simulink model "test_sliding_formation_gazebo_aerospace23a"  (R2023a)
settings: Solver=FixedStepAuto  StartTime=0.0  StopTime=inf  RelTol=1e-3
undefined symbols (not defined in the file or in its folder): angular, DiscIntNeverNeededParam, linear
libraries: ros2lib x11, simulink x4, robotcorelib x4
(part 1 of 2)
settings Model: Creator=johvany  LastModifiedBy=l15
settings OptimizationCC: EnhancedBackFolding=on  PassReuseOutputArgsThreshold=0  MaxStackSize=64  OptimizeBlockOrder=speed  DifferentSizesBufferReuse=on  OptimizationCustomize=off
settings DebuggingCC: ParameterTunabilityLossMsg=error
settings HardwareCC: ProdBitPerLong=64  ProdHWDeviceType=Intel->x86-64 (Linux 64)  UseEmbeddedCoderFeatures=off
settings SFSimCC: MATLABDynamicMemAlloc=off
settings RTWCC: Description=Simulink Desktop Real-Time  SystemTargetFile=sldrt.tlc  TemplateMakefile=sldrt.tmf  Toolchain=Colcon Tools  RTWCompilerOptimization=on
settings CodeAppCC: ForceParamTrailComments=on  MaxIdLength=95  OperatorAnnotations=on
settings SimulinkDesktopRealTimeCC: TargetLibSuffix=_sldrt.a  TargetPreCompLibLocation=/usr/local/MATLAB/R2023b/toolbox/sldrt/lib/glnxa64  TargetLangStandard=C89/C90 (ANSI)

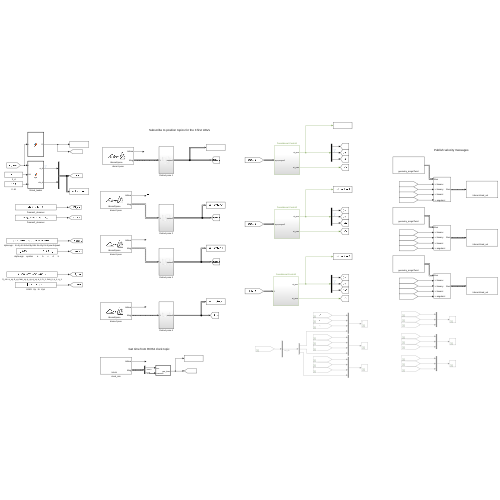
[thumbnail: Simulink's stored preview of the top-level diagram]
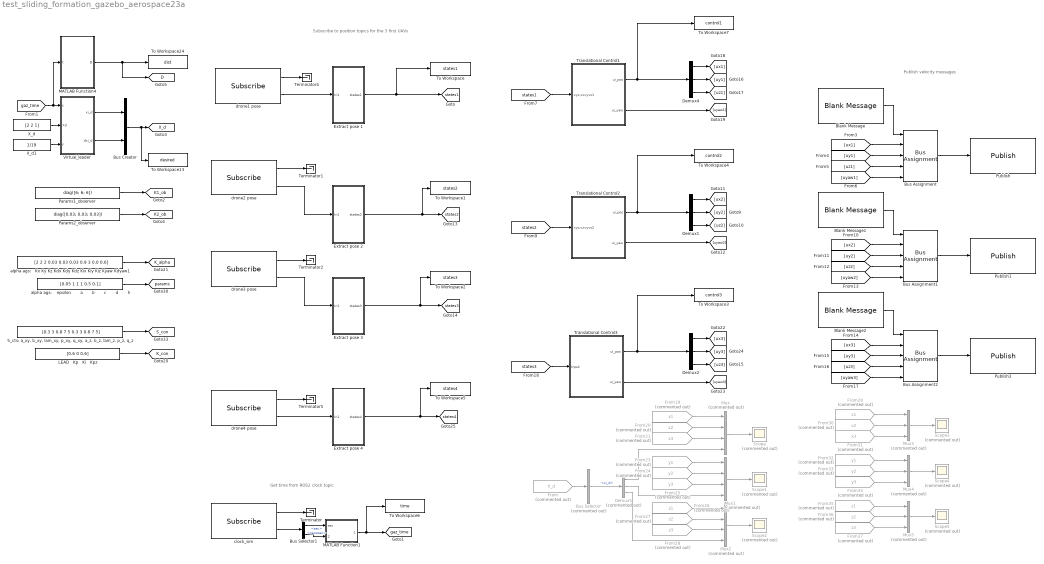
== system test_sliding_formation_gazebo_aerospace23a ==
  note: Publish velocity messages
  note: Subscribe to position topics for the 3 first UAVs
  note: Get time from ROS2 clock topic
  Blank Message : ros2lib/Blank Message  messageClass=Message  entityType=geometry_msgs/Twist  messageType=geometry_msgs/Twist  SampleTime=inf
  Blank Message1 : ros2lib/Blank Message  messageClass=Message  entityType=geometry_msgs/Twist  messageType=geometry_msgs/Twist  SampleTime=inf
  Blank Message2 : ros2lib/Blank Message  messageClass=Message  entityType=geometry_msgs/Twist  messageType=geometry_msgs/Twist  SampleTime=inf
  Bus Assignment : BusAssignment  AssignedSignals=linear.x,linear.y,linear.z,angular.z
  Bus Assignment1 : BusAssignment  AssignedSignals=linear.x,linear.y,linear.z,angular.z
  Bus Assignment2 : BusAssignment  AssignedSignals=linear.x,linear.y,linear.z,angular.z
  Bus Creator : BusCreator  Inputs=2
  Bus Selector : BusSelector  Commented=on  OutputSignals=xi_d
  Bus Selector1 : BusSelector  OutputSignals=clock.sec,clock.nanosec
  Demux1 : Demux  Outputs=3
  Demux2 : Demux  Outputs=3
  Demux4 : Demux  Outputs=3
  Demux5 : Demux  Commented=on  Outputs=3
  Extract pose 1 : Subsystem
  Extract pose 2 : Subsystem
  Extract pose 3 : Subsystem
  Extract pose 4 : Subsystem
  From : From  Commented=on  GotoTag=X_d  TagVisibility=global
      settings: CloseFcn=tagdialog Close
  From19 : From  Commented=on  GotoTag=x1  TagVisibility=global
      settings: CloseFcn=tagdialog Close
  From20 : From  Commented=on  GotoTag=x2  TagVisibility=global
      settings: CloseFcn=tagdialog Close
  From21 : From  Commented=on  GotoTag=x3  TagVisibility=global
      settings: CloseFcn=tagdialog Close
  From23 : From  Commented=on  GotoTag=y1  TagVisibility=global
      settings: CloseFcn=tagdialog Close
  From24 : From  Commented=on  GotoTag=y2  TagVisibility=global
      settings: CloseFcn=tagdialog Close
  From25 : From  Commented=on  GotoTag=y3  TagVisibility=global
      settings: CloseFcn=tagdialog Close
  From26 : From  Commented=on  GotoTag=z1  TagVisibility=global
      settings: CloseFcn=tagdialog Close
  From27 : From  Commented=on  GotoTag=z2  TagVisibility=global
      settings: CloseFcn=tagdialog Close
  From28 : From  Commented=on  GotoTag=z3  TagVisibility=global
      settings: CloseFcn=tagdialog Close
  From29 : From  Commented=on  GotoTag=x1  TagVisibility=global
      settings: CloseFcn=tagdialog Close
  From30 : From  Commented=on  GotoTag=x2  TagVisibility=global
      settings: CloseFcn=tagdialog Close
  From31 : From  Commented=on  GotoTag=x3  TagVisibility=global
      settings: CloseFcn=tagdialog Close
  From32 : From  Commented=on  GotoTag=y1  TagVisibility=global
      settings: CloseFcn=tagdialog Close
  From33 : From  Commented=on  GotoTag=y2  TagVisibility=global
      settings: CloseFcn=tagdialog Close
  From34 : From  Commented=on  GotoTag=y3  TagVisibility=global
      settings: CloseFcn=tagdialog Close
  From35 : From  Commented=on  GotoTag=z1  TagVisibility=global
      settings: CloseFcn=tagdialog Close
  From36 : From  Commented=on  GotoTag=z2  TagVisibility=global
      settings: CloseFcn=tagdialog Close
  From37 : From  Commented=on  GotoTag=z3  TagVisibility=global
      settings: CloseFcn=tagdialog Close
  LEAD   Kp   Ki   Kpz : Constant  Value=[0.6 0 0.6]
  MATLAB Function1 : MATLAB Function  TreatAsAtomicUnit=on
  MATLAB Function4 : MATLAB Function  TreatAsAtomicUnit=on
  Mux : Mux  Commented=on
  Mux1 : Mux  Commented=on
  Mux2 : Mux  Commented=on
  Mux3 : Mux  Commented=on  Inputs=3
  Mux4 : Mux  Commented=on  Inputs=3
  Mux5 : Mux  Commented=on  Inputs=3
  Params1_observer : Constant  Value=diag([6; 6; 6])
  Params2_observer : Constant  Value=diag([0.03; 0.03; 0.03])
  Publish : ros2lib/Publish  topicSource=Select from ROS network  topic=/drone1/cmd_vel  messageType=geometry_msgs/Twist  QOSHistory=Keep last  QOSDepth=1  QOSReliability=Reliable  QOSDurability=Volatile
  Publish1 : ros2lib/Publish  topicSource=Select from ROS network  topic=/drone2/cmd_vel  messageType=geometry_msgs/Twist  QOSHistory=Keep last  QOSDepth=1  QOSReliability=Reliable  QOSDurability=Volatile
  Publish2 : ros2lib/Publish  topicSource=Select from ROS network  topic=/drone3/cmd_vel  messageType=geometry_msgs/Twist  QOSHistory=Keep last  QOSDepth=1  QOSReliability=Reliable  QOSDurability=Volatile
  "S_cts: a_xy, b_xy, lam_xy, p_xy, q_xy, a_z, b_z, lam_z, p_z, q_z" : Constant  Value=[0.3 3 0.8 7 5 0.3 3 0.8 7 5]
  Scope{,1..5} (6 alike) : Scope  Commented=on
  Terminator{,1..2,4..5} (5 alike) : Terminator
  To Workspace : ToWorkspace  VariableName=states1  SampleTime=-1
  To Workspace1 : ToWorkspace  VariableName=states2  SampleTime=-1
  To Workspace13 : ToWorkspace  VariableName=desired  SampleTime=-1
  To Workspace2 : ToWorkspace  VariableName=states3  SampleTime=-1
  To Workspace24 : ToWorkspace  VariableName=dist  SampleTime=-1
  To Workspace3 : ToWorkspace  VariableName=control3  SampleTime=-1
  To Workspace4 : ToWorkspace  VariableName=control2  SampleTime=-1
  To Workspace5 : ToWorkspace  VariableName=states4  SampleTime=-1
  To Workspace6 : ToWorkspace  VariableName=time  SampleTime=-1
  To Workspace7 : ToWorkspace  VariableName=control1  SampleTime=-1
  Translational Control1 : Subsystem
  Translational Control2 : Subsystem
  Translational Control3 : Subsystem
  Virtual_leader : MATLAB Function  TreatAsAtomicUnit=on
  X_d : Constant  Value=[2 2 1]
  X_d1 : Constant  Value=1/19
  alpha ags:    epsilon       a       b       c       d       h : Constant  Value=[0.05 1 1 1 0.5 0.1]
  alpha ags:   Kx Ky Kz Kdx Kdy Kdz Kix Kiy Kiz Kyaw Kdyaw1 : Constant  Value=[2 2 2 0.03 0.03 0.03 0.9 3 0.0 0.6]
  clock_sim : ros2lib/Subscribe  topicSource=Select from ROS network  topic=/clock  messageType=rosgraph_msgs/Clock  sampleTime=-1  QOSHistory=Keep last  QOSDepth=1  QOSReliability=Reliable  QOSDurability=Volatile
  drone1 pose : ros2lib/Subscribe  topicSource=Select from ROS network  topic=/drone1/pose  messageType=geometry_msgs/PoseStamped  sampleTime=-1  QOSHistory=Keep last  QOSDepth=1  QOSReliability=Reliable  QOSDurability=Volatile
  drone2 pose : ros2lib/Subscribe  topicSource=Select from ROS network  topic=/drone2/pose  messageType=geometry_msgs/PoseStamped  sampleTime=-1  QOSHistory=Keep last  QOSDepth=1  QOSReliability=Reliable  QOSDurability=Volatile
  drone3 pose : ros2lib/Subscribe  topicSource=Select from ROS network  topic=/drone3/pose  messageType=geometry_msgs/PoseStamped  sampleTime=-1  QOSHistory=Keep last  QOSDepth=1  QOSReliability=Reliable  QOSDurability=Volatile
  drone4 pose : ros2lib/Subscribe  topicSource=Select from ROS network  topic=/drone4/pose  messageType=geometry_msgs/PoseStamped  sampleTime=-1  QOSHistory=Keep last  QOSDepth=1  QOSReliability=Reliable  QOSDurability=Volatile
  tag scope: D=global, K1_ob=global, K2_ob=global, K_alpha=global, K_con=global, S_con=global, X_d=global, gaz_time=global, params=global, states1=global, states2=global, states3=global, states4=global
  wires:
  clock_sim/1 -> Terminator/1
  drone2 pose/2 -> Extract pose 2/1(In1)
  drone2 pose/1 -> Terminator1/1
  drone3 pose/2 -> Extract pose 3/1(In1)
  drone3 pose/1 -> Terminator2/1
  Blank Message/1 -> Bus Assignment/1
  Bus Assignment/1 -> Publish/1
  Blank Message1/1 -> Bus Assignment1/1
  Bus Assignment1/1 -> Publish1/1
  Blank Message2/1 -> Bus Assignment2/1
  Bus Assignment2/1 -> Publish2/1
  clock_sim/2 -> Bus Selector1/1
  Bus Selector1/1 -> MATLAB Function1/1(sec)  "<sec>"
  Bus Selector1/2 -> MATLAB Function1/2(nanosec)  "<nanosec>"
  Virtual_leader/2(dxi_d) -> Bus Creator/2
  Bus Creator/1 -> To Workspace13/1, [X_d]
  Virtual_leader/1(xi_d) -> Bus Creator/1
  drone1 pose/1 -> Terminator4/1
  drone1 pose/2 -> Extract pose 1/1(In1)
  MATLAB Function1/1(gaz_time) -> To Workspace6/1, [gaz_time]
  Extract pose 1/1(states1) -> To Workspace/1, [states1]
  [ux1] -> Bus Assignment/2
  [uy1] -> Bus Assignment/3
  [uz1] -> Bus Assignment/4
  [uyaw1] -> Bus Assignment/5
  X_d/1 -> Virtual_leader/2(Xd)
  Extract pose 2/1(states2) -> To Workspace1/1, [states2]
  Extract pose 3/1(states3) -> To Workspace2/1, [states3]
  [ux2] -> Bus Assignment1/2
  [uy2] -> Bus Assignment1/3
  [uz2] -> Bus Assignment1/4
  [uyaw2] -> Bus Assignment1/5
  [uy3] -> Bus Assignment2/3
  [uyaw3] -> Bus Assignment2/5
  [uz3] -> Bus Assignment2/4
  [ux3] -> Bus Assignment2/2
  Translational Control1/2(ui_yaw) -> [uyaw1]
  Demux4/2 -> [uy1]
  Demux4/3 -> [uz1]
  [states1] -> Translational Control1/1(xyz,vxvyvz1)
  Demux4/1 -> [ux1]
  LEAD   Kp   Ki   Kpz/1 -> [K_con]
  alpha ags:   Kx Ky Kz Kdx Kdy Kdz Kix Kiy Kiz Kyaw Kdyaw1/1 -> [K_alpha]
  alpha ags:    epsilon       a       b       c       d       h/1 -> [params]
  X_d1/1 -> Virtual_leader/3(f)
  "S_cts: a_xy, b_xy, lam_xy, p_xy, q_xy, a_z, b_z, lam_z, p_z, q_z"/1 -> [S_con]
  MATLAB Function4/1(D) -> [D], To Workspace24/1
  [gaz_time] -> MATLAB Function4/1(t), Virtual_leader/1(t)
  Translational Control1/1(ui_pos) -> Demux4/1, To Workspace7/1
  Params1_observer/1 -> [K1_ob]
  Params2_observer/1 -> [K2_ob]
  Translational Control2/1(ui_pos) -> Demux1/1, To Workspace4/1
  Demux1/1 -> [ux2]
  [states2] -> Translational Control2/1(xyz,vxvyvz2)
  Demux1/3 -> [uz2]
  Demux1/2 -> [uy2]
  Translational Control2/2(ui_yaw) -> [uyaw2]
  Translational Control3/2(ui_yaw) -> [uyaw3]
  Demux2/2 -> [uy3]
  Demux2/3 -> [uz3]
  [states3] -> Translational Control3/1(Input)
  Demux2/1 -> [ux3]
  Translational Control3/1(ui_pos) -> Demux2/1, To Workspace3/1
  Extract pose 4/1(states4) -> [states4], To Workspace5/1
  drone4 pose/1 -> Terminator5/1
  drone4 pose/2 -> Extract pose 4/1(In1)
  From19/1 -> Mux/1
  From20/1 -> Mux/2
  From21/1 -> Mux/3
  Mux/1 -> Scope/1
  Bus Selector/1 -> Demux5/1  "<xi_d>"
  From/1 -> Bus Selector/1
  Demux5/1 -> Mux/4
  Demux5/2 -> Mux1/4
  Mux1/1 -> Scope1/1
  From25/1 -> Mux1/3
  From24/1 -> Mux1/2
  From23/1 -> Mux1/1
  From26/1 -> Mux2/1
  From27/1 -> Mux2/2
  From28/1 -> Mux2/3
  Mux2/1 -> Scope2/1
  Demux5/3 -> Mux2/4
  Mux5/1 -> Scope5/1
  From37/1 -> Mux5/3
  From36/1 -> Mux5/2
  From35/1 -> Mux5/1
  From32/1 -> Mux4/1
  From33/1 -> Mux4/2
  From34/1 -> Mux4/3
  Mux4/1 -> Scope4/1
  Mux3/1 -> Scope3/1
  From31/1 -> Mux3/3
  From30/1 -> Mux3/2
  From29/1 -> Mux3/1

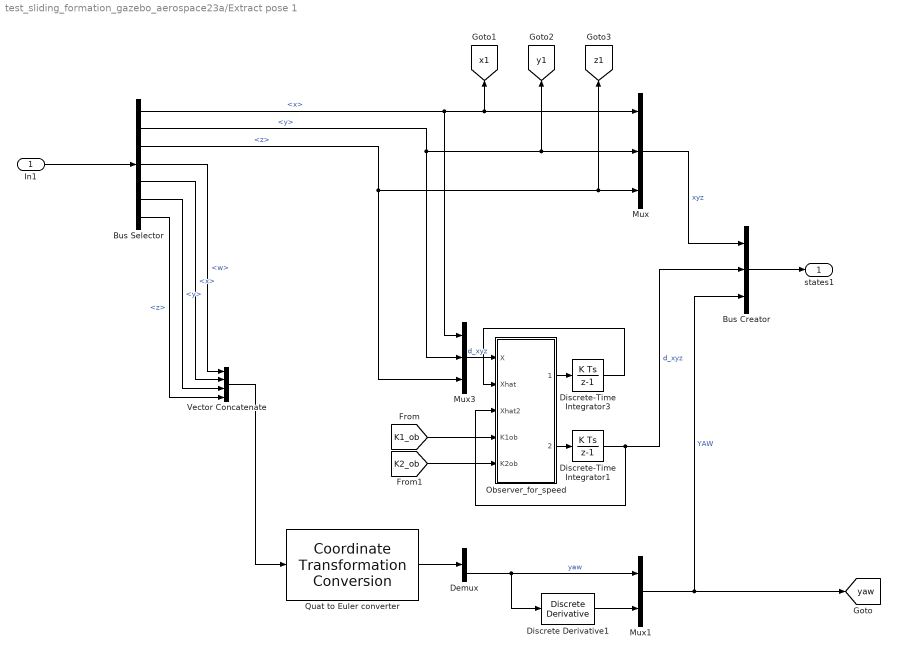
== system test_sliding_formation_gazebo_aerospace23a/Extract pose 1 ==
  In1 : Inport
  Bus Creator : BusCreator  Inputs=3
  Bus Selector : BusSelector  OutputSignals=pose.position.x,pose.position.y,pose.position.z,pose.orientation.w,pose.orientation.x,pose.orientation.y,pose.orientation.z
  Demux : Demux  Outputs=3
  Discrete Derivative1 : simulink/Discrete/Discrete Derivative  gainval=1.0  ICPrevScaledInput=0.0  OutMin=[]  OutMax=[]  OutDataType=fixdt(1, 16)  OutScaling=2^-10  DoSatur=off
  Discrete-Time Integrator1 : DiscreteIntegrator  SampleTime=-1  UpperSaturationLimit=1  LowerSaturationLimit=-1  ICPrevOutput=DiscIntNeverNeededParam  ICPrevScaledInput=DiscIntNeverNeededParam
  Discrete-Time Integrator3 : DiscreteIntegrator  SampleTime=-1  UpperSaturationLimit=1  LowerSaturationLimit=-1  ICPrevOutput=DiscIntNeverNeededParam  ICPrevScaledInput=DiscIntNeverNeededParam
  Mux : Mux  Inputs=3
  Mux1 : Mux  Inputs=2
  Mux3 : Mux  Inputs=3
  Observer_for_speed : MATLAB Function  TreatAsAtomicUnit=on
  Quat to Euler converter : robotcorelib/Coordinate Transformation Conversion  InputRepresentation=Quaternion  InputEulerSequence=ZYX  ShowTrVecInputPort=on  OutputRepresentation=Euler Angles  OutputEulerSequence=XYZ  ShowTrVecOutputPort=on  SimulateUsing=Interpreted execution
      settings: LibrarySourceBlock=roslib/Utilities/Coordinate Transformation Conversion
  Vector Concatenate : Concatenate  NumInputs=4
  states1 : Outport
  tag scope: x1=global, y1=global, yaw=global, z1=global
  wires:
  Bus Selector/5 -> Vector Concatenate/2  "<x>"
  Quat to Euler converter/1 -> Demux/1
  Bus Selector/6 -> Vector Concatenate/3  "<y>"
  Bus Selector/7 -> Vector Concatenate/4  "<z>"
  Vector Concatenate/1 -> Quat to Euler converter/1
  In1/1 -> Bus Selector/1
  Bus Selector/4 -> Vector Concatenate/1  "<w>"
  Demux/3 -> Discrete Derivative1/1, Mux1/1  "yaw"
  Mux/1 -> Bus Creator/1  "xyz"
  Bus Creator/1 -> states1/1
  Discrete Derivative1/1 -> Mux1/2
  Bus Selector/3 -> Mux3/3, [z1], Mux/3  "<z>"
  Bus Selector/2 -> Mux3/2, [y1], Mux/2  "<y>"
  Bus Selector/1 -> Mux3/1, [x1], Mux/1  "<x>"
  Mux1/1 -> [yaw], Bus Creator/3  "YAW"
  Discrete-Time Integrator1/1 -> Observer_for_speed/3(Xhat2), Bus Creator/2  "d_xyz"
  Discrete-Time Integrator3/1 -> Observer_for_speed/2(Xhat)
  Observer_for_speed/1(dXhat_1) -> Discrete-Time Integrator3/1
  Observer_for_speed/2(dXhat_2) -> Discrete-Time Integrator1/1
  Mux3/1 -> Observer_for_speed/1(X)  "d_xyz"
  [K1_ob] -> Observer_for_speed/4(K1ob)
  [K2_ob] -> Observer_for_speed/5(K2ob)

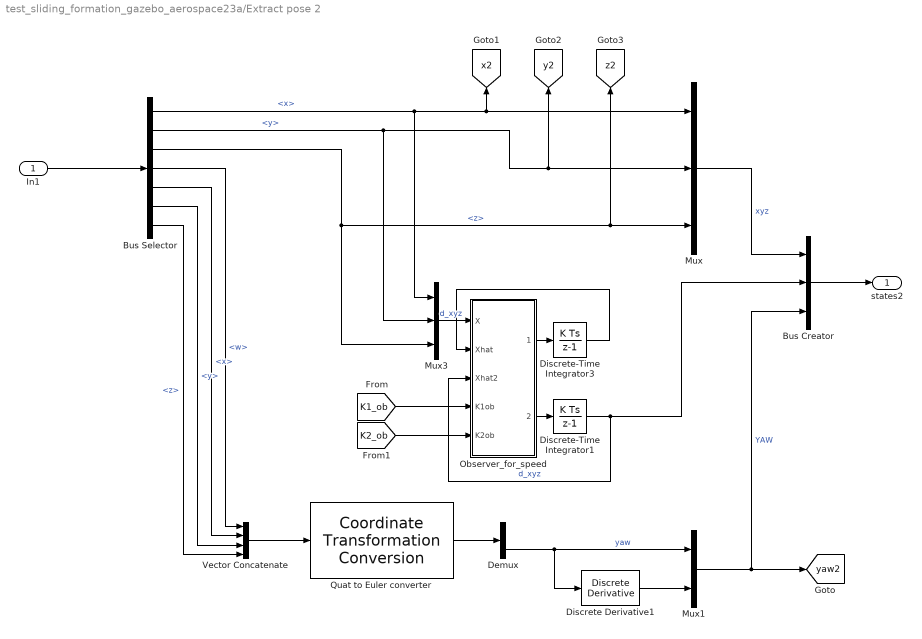
== system test_sliding_formation_gazebo_aerospace23a/Extract pose 2 ==
  In1 : Inport
  Bus Creator : BusCreator  Inputs=3
  Bus Selector : BusSelector  OutputSignals=pose.position.x,pose.position.y,pose.position.z,pose.orientation.w,pose.orientation.x,pose.orientation.y,pose.orientation.z
  Demux : Demux  Outputs=3
  Discrete Derivative1 : simulink/Discrete/Discrete Derivative  gainval=1.0  ICPrevScaledInput=0.0  OutMin=[]  OutMax=[]  OutDataType=fixdt(1, 16)  OutScaling=2^-10  DoSatur=off
  Discrete-Time Integrator1 : DiscreteIntegrator  SampleTime=-1  UpperSaturationLimit=1  LowerSaturationLimit=-1  ICPrevOutput=DiscIntNeverNeededParam  ICPrevScaledInput=DiscIntNeverNeededParam
  Discrete-Time Integrator3 : DiscreteIntegrator  SampleTime=-1  UpperSaturationLimit=1  LowerSaturationLimit=-1  ICPrevOutput=DiscIntNeverNeededParam  ICPrevScaledInput=DiscIntNeverNeededParam
  Mux : Mux  Inputs=3
  Mux1 : Mux  Inputs=2
  Mux3 : Mux  Inputs=3
  Observer_for_speed : MATLAB Function  TreatAsAtomicUnit=on
  Quat to Euler converter : robotcorelib/Coordinate Transformation Conversion  InputRepresentation=Quaternion  InputEulerSequence=ZYX  ShowTrVecInputPort=on  OutputRepresentation=Euler Angles  OutputEulerSequence=XYZ  ShowTrVecOutputPort=on  SimulateUsing=Interpreted execution
      settings: LibrarySourceBlock=roslib/Utilities/Coordinate Transformation Conversion
  Vector Concatenate : Concatenate  NumInputs=4
  states2 : Outport
  tag scope: x2=global, y2=global, yaw2=global, z2=global
  wires:
  Discrete Derivative1/1 -> Mux1/2
  Bus Creator/1 -> states2/1
  Mux/1 -> Bus Creator/1  "xyz"
  Demux/3 -> Discrete Derivative1/1, Mux1/1  "yaw"
  Bus Selector/4 -> Vector Concatenate/1  "<w>"
  In1/1 -> Bus Selector/1
  Vector Concatenate/1 -> Quat to Euler converter/1
  Bus Selector/7 -> Vector Concatenate/4  "<z>"
  Bus Selector/6 -> Vector Concatenate/3  "<y>"
  Quat to Euler converter/1 -> Demux/1
  Bus Selector/5 -> Vector Concatenate/2  "<x>"
  Mux3/1 -> Observer_for_speed/1(X)  "d_xyz"
  Observer_for_speed/1(dXhat_1) -> Discrete-Time Integrator3/1
  Observer_for_speed/2(dXhat_2) -> Discrete-Time Integrator1/1
  [K1_ob] -> Observer_for_speed/4(K1ob)
  Bus Selector/2 -> Mux3/2, [y2], Mux/2  "<y>"
  Bus Selector/1 -> Mux3/1, [x2], Mux/1  "<x>"
  Discrete-Time Integrator3/1 -> Observer_for_speed/2(Xhat)
  Discrete-Time Integrator1/1 -> Bus Creator/2, Observer_for_speed/3(Xhat2)  "d_xyz"
  [K2_ob] -> Observer_for_speed/5(K2ob)
  Bus Selector/3 -> Mux3/3, [z2], Mux/3  "<z>"
  Mux1/1 -> [yaw2], Bus Creator/3  "YAW"

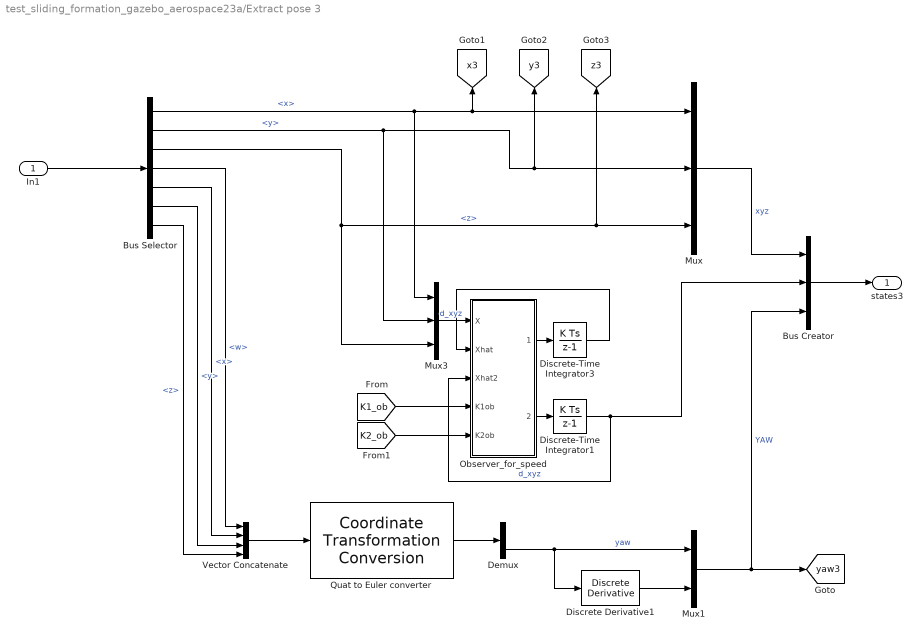
== system test_sliding_formation_gazebo_aerospace23a/Extract pose 3 ==
  In1 : Inport
  Bus Creator : BusCreator  Inputs=3
  Bus Selector : BusSelector  OutputSignals=pose.position.x,pose.position.y,pose.position.z,pose.orientation.w,pose.orientation.x,pose.orientation.y,pose.orientation.z
  Demux : Demux  Outputs=3
  Discrete Derivative1 : simulink/Discrete/Discrete Derivative  gainval=1.0  ICPrevScaledInput=0.0  OutMin=[]  OutMax=[]  OutDataType=fixdt(1, 16)  OutScaling=2^-10  DoSatur=off
  Discrete-Time Integrator1 : DiscreteIntegrator  SampleTime=-1  UpperSaturationLimit=1  LowerSaturationLimit=-1  ICPrevOutput=DiscIntNeverNeededParam  ICPrevScaledInput=DiscIntNeverNeededParam
  Discrete-Time Integrator3 : DiscreteIntegrator  SampleTime=-1  UpperSaturationLimit=1  LowerSaturationLimit=-1  ICPrevOutput=DiscIntNeverNeededParam  ICPrevScaledInput=DiscIntNeverNeededParam
  Mux : Mux  Inputs=3
  Mux1 : Mux  Inputs=2
  Mux3 : Mux  Inputs=3
  Observer_for_speed : MATLAB Function  TreatAsAtomicUnit=on
  Quat to Euler converter : robotcorelib/Coordinate Transformation Conversion  InputRepresentation=Quaternion  InputEulerSequence=ZYX  ShowTrVecInputPort=on  OutputRepresentation=Euler Angles  OutputEulerSequence=XYZ  ShowTrVecOutputPort=on  SimulateUsing=Interpreted execution
      settings: LibrarySourceBlock=roslib/Utilities/Coordinate Transformation Conversion
  Vector Concatenate : Concatenate  NumInputs=4
  states3 : Outport
  tag scope: x3=global, y3=global, yaw3=global, z3=global
  wires:
  Mux1/1 -> Bus Creator/3, [yaw3]  "YAW"
  Bus Selector/3 -> [z3], Mux/3, Mux3/3  "<z>"
  [K2_ob] -> Observer_for_speed/5(K2ob)
  Discrete-Time Integrator1/1 -> Observer_for_speed/3(Xhat2), Bus Creator/2  "d_xyz"
  Discrete-Time Integrator3/1 -> Observer_for_speed/2(Xhat)
  Bus Selector/1 -> [x3], Mux/1, Mux3/1  "<x>"
  Bus Selector/2 -> [y3], Mux/2, Mux3/2  "<y>"
  [K1_ob] -> Observer_for_speed/4(K1ob)
  Observer_for_speed/2(dXhat_2) -> Discrete-Time Integrator1/1
  Observer_for_speed/1(dXhat_1) -> Discrete-Time Integrator3/1
  Mux3/1 -> Observer_for_speed/1(X)  "d_xyz"
  Bus Selector/5 -> Vector Concatenate/2  "<x>"
  Quat to Euler converter/1 -> Demux/1
  Bus Selector/6 -> Vector Concatenate/3  "<y>"
  Bus Selector/7 -> Vector Concatenate/4  "<z>"
  Vector Concatenate/1 -> Quat to Euler converter/1
  In1/1 -> Bus Selector/1
  Bus Selector/4 -> Vector Concatenate/1  "<w>"
  Demux/3 -> Mux1/1, Discrete Derivative1/1  "yaw"
  Mux/1 -> Bus Creator/1  "xyz"
  Bus Creator/1 -> states3/1
  Discrete Derivative1/1 -> Mux1/2

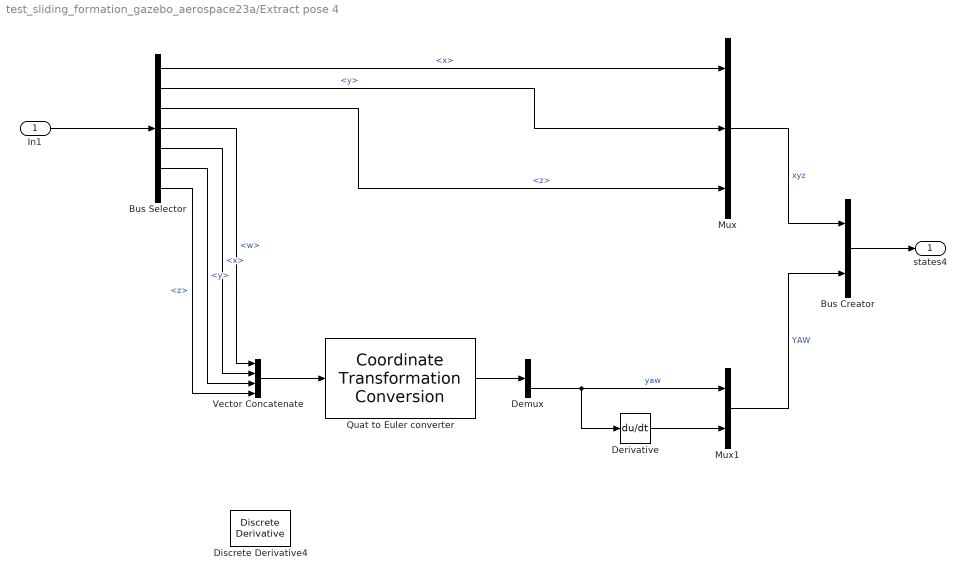
== system test_sliding_formation_gazebo_aerospace23a/Extract pose 4 ==
  In1 : Inport
  Bus Creator : BusCreator  Inputs=2
  Bus Selector : BusSelector  OutputSignals=pose.position.x,pose.position.y,pose.position.z,pose.orientation.w,pose.orientation.x,pose.orientation.y,pose.orientation.z
  Demux : Demux  Outputs=3
  Derivative : Derivative
  Discrete Derivative4 : simulink/Discrete/Discrete Derivative  gainval=1.0  ICPrevScaledInput=0.0  OutMin=[]  OutMax=[]  OutDataType=fixdt(1, 16)  OutScaling=2^-10  DoSatur=off
  Mux : Mux  Inputs=3
  Mux1 : Mux  Inputs=2
  Quat to Euler converter : robotcorelib/Coordinate Transformation Conversion  InputRepresentation=Quaternion  InputEulerSequence=ZYX  ShowTrVecInputPort=on  OutputRepresentation=Euler Angles  OutputEulerSequence=XYZ  ShowTrVecOutputPort=on  SimulateUsing=Interpreted execution
      settings: LibrarySourceBlock=roslib/Utilities/Coordinate Transformation Conversion
  Vector Concatenate : Concatenate  NumInputs=4
  states4 : Outport
  wires:
  Bus Selector/5 -> Vector Concatenate/2  "<x>"
  Quat to Euler converter/1 -> Demux/1
  Bus Selector/6 -> Vector Concatenate/3  "<y>"
  Bus Selector/1 -> Mux/1  "<x>"
  Bus Selector/7 -> Vector Concatenate/4  "<z>"
  Vector Concatenate/1 -> Quat to Euler converter/1
  In1/1 -> Bus Selector/1
  Bus Selector/4 -> Vector Concatenate/1  "<w>"
  Bus Selector/2 -> Mux/2  "<y>"
  Bus Selector/3 -> Mux/3  "<z>"
  Demux/3 -> Derivative/1, Mux1/1  "yaw"
  Mux/1 -> Bus Creator/1  "xyz"
  Bus Creator/1 -> states4/1
  Derivative/1 -> Mux1/2
  Mux1/1 -> Bus Creator/2  "YAW"

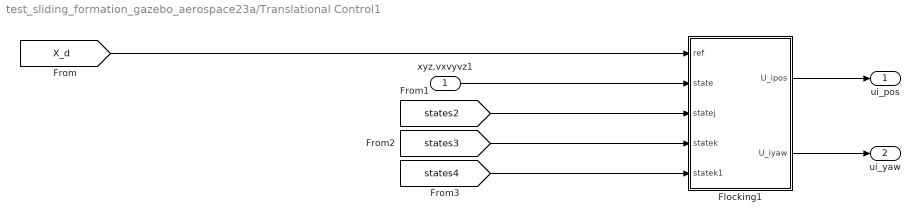
== system test_sliding_formation_gazebo_aerospace23a/Translational Control1 ==
  xyz,vxvyvz1 : Inport
  Flocking1 : Subsystem
  ui_pos : Outport  VectorParamsAs1DForOutWhenUnconnected=off
  ui_yaw : Outport  Port=2  VectorParamsAs1DForOutWhenUnconnected=off
  wires:
  [states2] -> Flocking1/3(statej)
  [states3] -> Flocking1/4(statek)
  [states4] -> Flocking1/5(statek1)
  Flocking1/1(U_ipos) -> ui_pos/1
  Flocking1/2(U_iyaw) -> ui_yaw/1
  [X_d] -> Flocking1/1(ref)
  xyz,vxvyvz1/1 -> Flocking1/2(state)

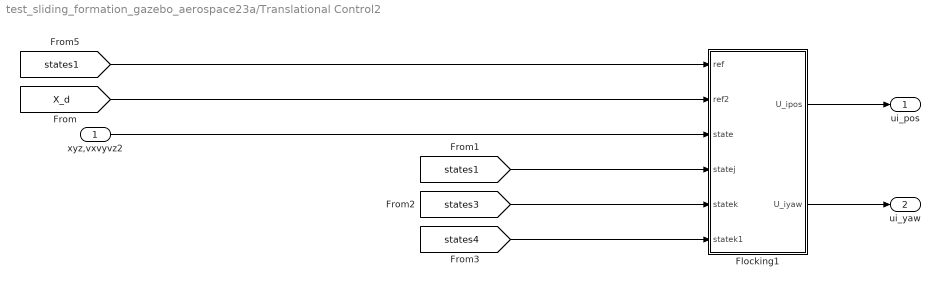
== system test_sliding_formation_gazebo_aerospace23a/Translational Control2 ==
  xyz,vxvyvz2 : Inport
  Flocking1 : Subsystem
  ui_pos : Outport  VectorParamsAs1DForOutWhenUnconnected=off
  ui_yaw : Outport  Port=2  VectorParamsAs1DForOutWhenUnconnected=off
  wires:
  Flocking1/2(U_iyaw) -> ui_yaw/1
  Flocking1/1(U_ipos) -> ui_pos/1
  [states4] -> Flocking1/6(statek1)
  [states3] -> Flocking1/5(statek)
  [states1] -> Flocking1/4(statej)
  [states1] -> Flocking1/1(ref)
  [X_d] -> Flocking1/2(ref2)
  xyz,vxvyvz2/1 -> Flocking1/3(state)

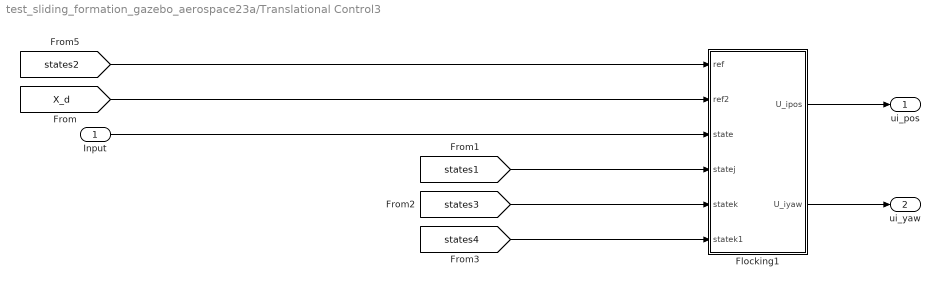
== system test_sliding_formation_gazebo_aerospace23a/Translational Control3 ==
  Input : Inport
  Flocking1 : Subsystem
  ui_pos : Outport  VectorParamsAs1DForOutWhenUnconnected=off
  ui_yaw : Outport  Port=2  VectorParamsAs1DForOutWhenUnconnected=off
  wires:
  [X_d] -> Flocking1/2(ref2)
  [states2] -> Flocking1/1(ref)
  [states1] -> Flocking1/4(statej)
  [states3] -> Flocking1/5(statek)
  [states4] -> Flocking1/6(statek1)
  Flocking1/1(U_ipos) -> ui_pos/1
  Flocking1/2(U_iyaw) -> ui_yaw/1
  Input/1 -> Flocking1/3(state)

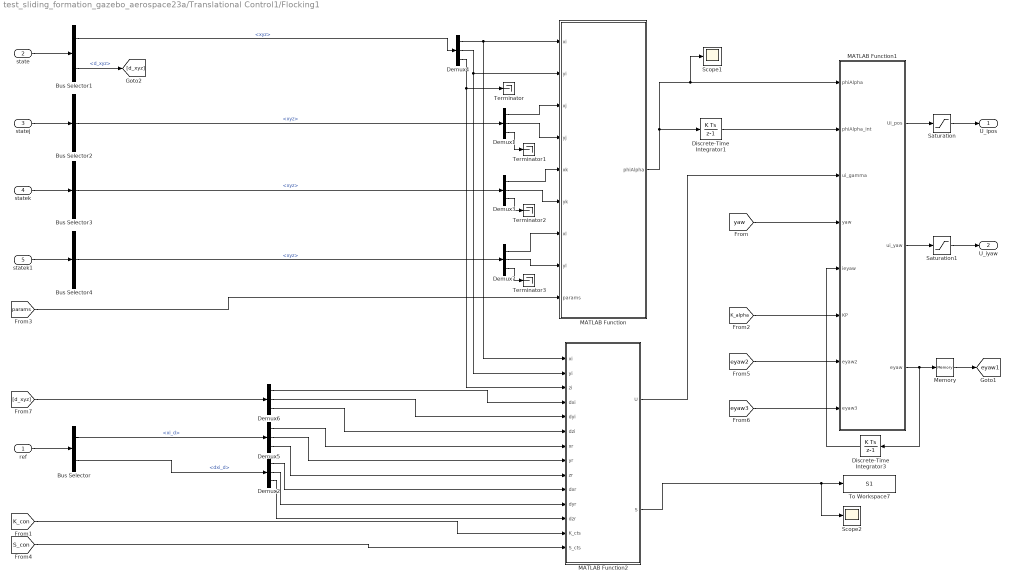
== system test_sliding_formation_gazebo_aerospace23a/Translational Control1/Flocking1 ==
  ref : Inport
  state : Inport  Port=2
  statej : Inport  Port=3
  statek : Inport  Port=4
  statek1 : Inport  Port=5
  Bus Selector : BusSelector  OutputSignals=xi_d,dxi_d
  Bus Selector1 : BusSelector  OutputSignals=xyz,d_xyz
  Bus Selector2 : BusSelector  OutputSignals=xyz
  Bus Selector3 : BusSelector  OutputSignals=xyz
  Bus Selector4 : BusSelector  OutputSignals=xyz
  Demux{1..7} (7 alike) : Demux  Outputs=3
  Discrete-Time Integrator1 : DiscreteIntegrator  SampleTime=-1  LimitOutput=on  UpperSaturationLimit=5  LowerSaturationLimit=-5  ICPrevOutput=DiscIntNeverNeededParam  ICPrevScaledInput=DiscIntNeverNeededParam
  Discrete-Time Integrator3 : DiscreteIntegrator  SampleTime=-1  LimitOutput=on  UpperSaturationLimit=1  LowerSaturationLimit=-1  ICPrevOutput=DiscIntNeverNeededParam  ICPrevScaledInput=DiscIntNeverNeededParam
  MATLAB Function : MATLAB Function  TreatAsAtomicUnit=on
  MATLAB Function1 : MATLAB Function  TreatAsAtomicUnit=on
  MATLAB Function2 : MATLAB Function  TreatAsAtomicUnit=on
  Memory : Memory
  Saturation : Saturate  UpperLimit=1  LowerLimit=-1
  Saturation1 : Saturate  UpperLimit=1  LowerLimit=-1
  Scope1 : Scope
  Scope2 : Scope
  Terminator{,1..3} (4 alike) : Terminator
  To Workspace7 : ToWorkspace  VariableName=S1  SampleTime=-1
  U_ipos : Outport  VectorParamsAs1DForOutWhenUnconnected=off
  U_iyaw : Outport  Port=2  VectorParamsAs1DForOutWhenUnconnected=off
  tag scope: eyaw1=global
  wires:
  ref/1 -> Bus Selector/1
  state/1 -> Bus Selector1/1
  Bus Selector/1 -> Demux5/1  "<xi_d>"
  statej/1 -> Bus Selector2/1
  Bus Selector2/1 -> Demux1/1  "<xyz>"
  Demux4/1 -> MATLAB Function2/1(xi), MATLAB Function/1(xi)
  Demux4/2 -> MATLAB Function2/2(yi), MATLAB Function/2(yi)
  Demux1/1 -> MATLAB Function/3(xj)
  Demux1/2 -> MATLAB Function/4(yj)
  Discrete-Time Integrator1/1 -> MATLAB Function1/2(phiAlpha_int)
  MATLAB Function2/1(U) -> MATLAB Function1/3(ui_gamma)
  statek/1 -> Bus Selector3/1
  Demux3/1 -> MATLAB Function/5(xk)
  Demux3/2 -> MATLAB Function/6(yk)
  Bus Selector3/1 -> Demux3/1  "<xyz>"
  MATLAB Function/1(phiAlpha) -> Scope1/1, MATLAB Function1/1(phiAlpha), Discrete-Time Integrator1/1
  Demux5/1 -> MATLAB Function2/7(xr)
  Demux5/2 -> MATLAB Function2/8(yr)
  Demux4/3 -> Terminator/1, MATLAB Function2/3(zi)
  Demux3/3 -> Terminator2/1
  Demux5/3 -> MATLAB Function2/9(zr)
  MATLAB Function1/1(Ui_pos) -> Saturation/1
  Demux1/3 -> Terminator1/1
  statek1/1 -> Bus Selector4/1
  Demux7/1 -> MATLAB Function/7(xl)
  Demux7/2 -> MATLAB Function/8(yl)
  Demux7/3 -> Terminator3/1
  Bus Selector4/1 -> Demux7/1  "<xyz>"
  Bus Selector1/1 -> Demux4/1  "<xyz>"
  [yaw] -> MATLAB Function1/4(yaw)
  MATLAB Function1/2(ui_yaw) -> Saturation1/1
  [K_con] -> MATLAB Function2/13(K_cts)
  MATLAB Function1/3(eyaw) -> Discrete-Time Integrator3/1, Memory/1
  [K_alpha] -> MATLAB Function1/6(KP)
  [params] -> MATLAB Function/9(params)
  [S_con] -> MATLAB Function2/14(S_cts)
  Bus Selector/2 -> Demux2/1  "<dxi_d>"
  Demux2/1 -> MATLAB Function2/10(dxr)
  Demux2/2 -> MATLAB Function2/11(dyr)
  Demux2/3 -> MATLAB Function2/12(dzr)
  [eyaw2] -> MATLAB Function1/7(eyaw2)
  [eyaw3] -> MATLAB Function1/8(eyaw3)
  Memory/1 -> [eyaw1]
  Discrete-Time Integrator3/1 -> MATLAB Function1/5(ieyaw)
  MATLAB Function2/2(S) -> Scope2/1, To Workspace7/1
  Saturation/1 -> U_ipos/1
  Saturation1/1 -> U_iyaw/1
  Bus Selector1/2 -> [d_xyz]  "<d_xyz>"
  Demux6/1 -> MATLAB Function2/4(dxi)
  Demux6/2 -> MATLAB Function2/5(dyi)
  Demux6/3 -> MATLAB Function2/6(dzi)
  [d_xyz] -> Demux6/1

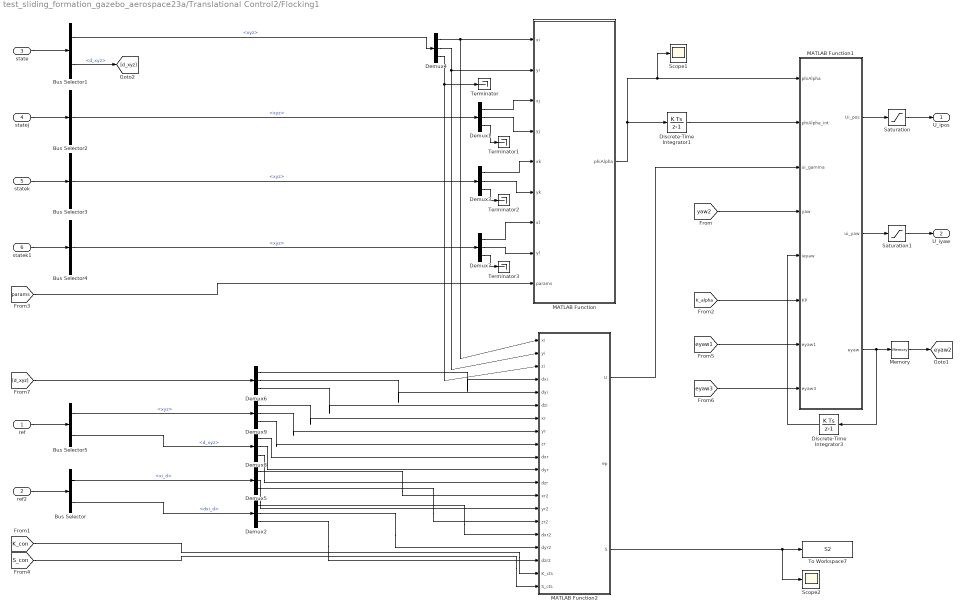
== system test_sliding_formation_gazebo_aerospace23a/Translational Control2/Flocking1 ==
  ref : Inport
  ref2 : Inport  Port=2
  state : Inport  Port=3
  statej : Inport  Port=4
  statek : Inport  Port=5
  statek1 : Inport  Port=6
  Bus Selector : BusSelector  OutputSignals=xi_d,dxi_d
  Bus Selector1 : BusSelector  OutputSignals=xyz,d_xyz
  Bus Selector2 : BusSelector  OutputSignals=xyz
  Bus Selector3 : BusSelector  OutputSignals=xyz
  Bus Selector4 : BusSelector  OutputSignals=xyz
  Bus Selector5 : BusSelector  OutputSignals=xyz,d_xyz
  Demux{1..9} (9 alike) : Demux  Outputs=3
  Discrete-Time Integrator1 : DiscreteIntegrator  SampleTime=-1  LimitOutput=on  UpperSaturationLimit=5  LowerSaturationLimit=-5  ICPrevOutput=DiscIntNeverNeededParam  ICPrevScaledInput=DiscIntNeverNeededParam
  Discrete-Time Integrator3 : DiscreteIntegrator  SampleTime=-1  LimitOutput=on  UpperSaturationLimit=1  LowerSaturationLimit=-1  ICPrevOutput=DiscIntNeverNeededParam  ICPrevScaledInput=DiscIntNeverNeededParam
  MATLAB Function : MATLAB Function  TreatAsAtomicUnit=on
  MATLAB Function1 : MATLAB Function  TreatAsAtomicUnit=on
  MATLAB Function2 : MATLAB Function  TreatAsAtomicUnit=on
  Memory : Memory
  Saturation : Saturate  UpperLimit=1  LowerLimit=-1
  Saturation1 : Saturate  UpperLimit=1  LowerLimit=-1
  Scope1 : Scope
  Scope2 : Scope
  Terminator{,1..3} (4 alike) : Terminator
  To Workspace7 : ToWorkspace  VariableName=S2  SampleTime=-1
  U_ipos : Outport  VectorParamsAs1DForOutWhenUnconnected=off
  U_iyaw : Outport  Port=2  VectorParamsAs1DForOutWhenUnconnected=off
  tag scope: eyaw2=global
  wires:
  [d_xyz] -> Demux6/1
  Demux6/3 -> MATLAB Function2/6(dzi)
  Demux6/2 -> MATLAB Function2/5(dyi)
  Demux6/1 -> MATLAB Function2/4(dxi)
  Bus Selector1/2 -> [d_xyz]  "<d_xyz>"
  Saturation1/1 -> U_iyaw/1
  Saturation/1 -> U_ipos/1
  MATLAB Function2/3(S) -> To Workspace7/1, Scope2/1
  Discrete-Time Integrator3/1 -> MATLAB Function1/5(ieyaw)
  Memory/1 -> [eyaw2]
  [eyaw3] -> MATLAB Function1/8(eyaw3)
  [eyaw1] -> MATLAB Function1/7(eyaw1)
  Bus Selector/2 -> Demux2/1  "<dxi_d>"
  [S_con] -> MATLAB Function2/20(S_cts)
  [params] -> MATLAB Function/9(params)
  [K_alpha] -> MATLAB Function1/6(KP)
  MATLAB Function1/3(eyaw) -> Memory/1, Discrete-Time Integrator3/1
  [K_con] -> MATLAB Function2/19(K_cts)
  MATLAB Function1/2(ui_yaw) -> Saturation1/1
  [yaw2] -> MATLAB Function1/4(yaw)
  Bus Selector1/1 -> Demux4/1  "<xyz>"
  Bus Selector4/1 -> Demux7/1  "<xyz>"
  Demux7/3 -> Terminator3/1
  Demux7/2 -> MATLAB Function/8(yl)
  Demux7/1 -> MATLAB Function/7(xl)
  statek1/1 -> Bus Selector4/1
  Demux1/3 -> Terminator1/1
  MATLAB Function1/1(Ui_pos) -> Saturation/1
  Demux3/3 -> Terminator2/1
  Demux4/3 -> MATLAB Function2/3(zi), Terminator/1
  MATLAB Function/1(phiAlpha) -> Discrete-Time Integrator1/1, MATLAB Function1/1(phiAlpha), Scope1/1
  Bus Selector3/1 -> Demux3/1  "<xyz>"
  Demux3/2 -> MATLAB Function/6(yk)
  Demux3/1 -> MATLAB Function/5(xk)
  statek/1 -> Bus Selector3/1
  MATLAB Function2/1(U) -> MATLAB Function1/3(ui_gamma)
  Discrete-Time Integrator1/1 -> MATLAB Function1/2(phiAlpha_int)
  Demux1/2 -> MATLAB Function/4(yj)
  Demux1/1 -> MATLAB Function/3(xj)
  Demux4/2 -> MATLAB Function/2(yi), MATLAB Function2/2(yi)
  Demux4/1 -> MATLAB Function/1(xi), MATLAB Function2/1(xi)
  Bus Selector2/1 -> Demux1/1  "<xyz>"
  statej/1 -> Bus Selector2/1
  Bus Selector/1 -> Demux5/1  "<xi_d>"
  state/1 -> Bus Selector1/1
  ref2/1 -> Bus Selector/1
  ref/1 -> Bus Selector5/1
  Bus Selector5/1 -> Demux9/1  "<xyz>"
  Bus Selector5/2 -> Demux8/1  "<d_xyz>"
  Demux9/2 -> MATLAB Function2/8(yr)
  Demux8/2 -> MATLAB Function2/11(dyr)
  Demux9/1 -> MATLAB Function2/7(xr)
  Demux9/3 -> MATLAB Function2/9(zr)
  Demux8/1 -> MATLAB Function2/10(dxr)
  Demux8/3 -> MATLAB Function2/12(dzr)
  Demux5/1 -> MATLAB Function2/13(xr2)
  Demux5/2 -> MATLAB Function2/14(yr2)
  Demux5/3 -> MATLAB Function2/15(zr2)
  Demux2/1 -> MATLAB Function2/16(dxr2)
  Demux2/2 -> MATLAB Function2/17(dyr2)
  Demux2/3 -> MATLAB Function2/18(dzr2)

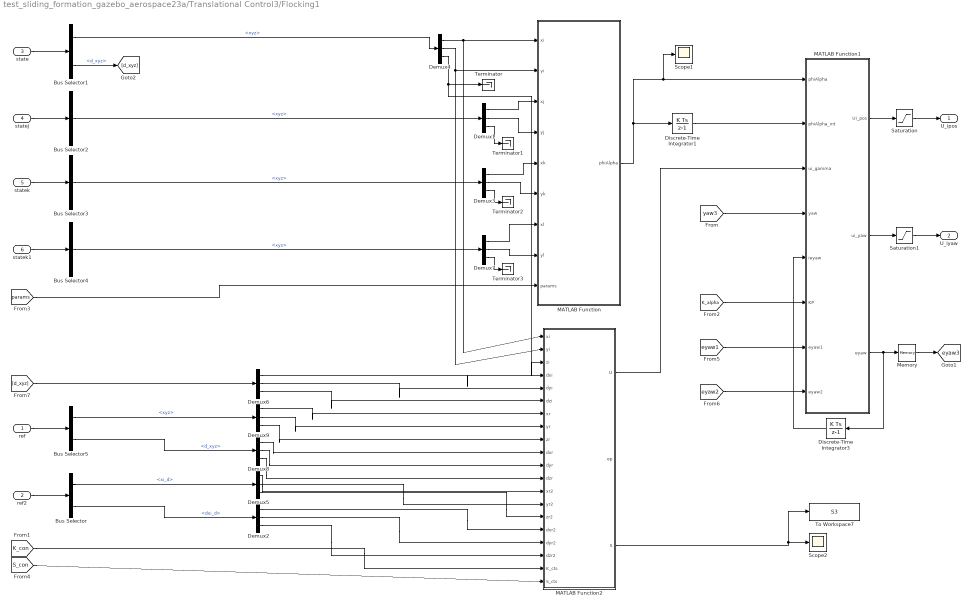
== system test_sliding_formation_gazebo_aerospace23a/Translational Control3/Flocking1 ==
  ref : Inport
  ref2 : Inport  Port=2
  state : Inport  Port=3
  statej : Inport  Port=4
  statek : Inport  Port=5
  statek1 : Inport  Port=6
  Bus Selector : BusSelector  OutputSignals=xi_d,dxi_d
  Bus Selector1 : BusSelector  OutputSignals=xyz,d_xyz
  Bus Selector2 : BusSelector  OutputSignals=xyz
  Bus Selector3 : BusSelector  OutputSignals=xyz
  Bus Selector4 : BusSelector  OutputSignals=xyz
  Bus Selector5 : BusSelector  OutputSignals=xyz,d_xyz
  Demux{1..9} (9 alike) : Demux  Outputs=3
  Discrete-Time Integrator1 : DiscreteIntegrator  SampleTime=-1  LimitOutput=on  UpperSaturationLimit=5  LowerSaturationLimit=-5  ICPrevOutput=DiscIntNeverNeededParam  ICPrevScaledInput=DiscIntNeverNeededParam
  Discrete-Time Integrator3 : DiscreteIntegrator  SampleTime=-1  LimitOutput=on  UpperSaturationLimit=1  LowerSaturationLimit=-1  ICPrevOutput=DiscIntNeverNeededParam  ICPrevScaledInput=DiscIntNeverNeededParam
  MATLAB Function : MATLAB Function  TreatAsAtomicUnit=on
  MATLAB Function1 : MATLAB Function  TreatAsAtomicUnit=on
  MATLAB Function2 : MATLAB Function  TreatAsAtomicUnit=on
  Memory : Memory
  Saturation : Saturate  UpperLimit=1  LowerLimit=-1
  Saturation1 : Saturate  UpperLimit=1  LowerLimit=-1
  Scope1 : Scope
  Scope2 : Scope
  Terminator{,1..3} (4 alike) : Terminator
  To Workspace7 : ToWorkspace  VariableName=S3  SampleTime=-1
  U_ipos : Outport  VectorParamsAs1DForOutWhenUnconnected=off
  U_iyaw : Outport  Port=2  VectorParamsAs1DForOutWhenUnconnected=off
  tag scope: eyaw3=global
  wires:
  Demux2/1 -> MATLAB Function2/16(dxr2)
  Demux5/1 -> MATLAB Function2/13(xr2)
  Demux2/2 -> MATLAB Function2/17(dyr2)
  Demux5/2 -> MATLAB Function2/14(yr2)
  Demux2/3 -> MATLAB Function2/18(dzr2)
  Demux5/3 -> MATLAB Function2/15(zr2)
  Demux8/3 -> MATLAB Function2/12(dzr)
  Demux8/1 -> MATLAB Function2/10(dxr)
  Demux9/3 -> MATLAB Function2/9(zr)
  Demux9/1 -> MATLAB Function2/7(xr)
  Demux8/2 -> MATLAB Function2/11(dyr)
  Demux9/2 -> MATLAB Function2/8(yr)
  Bus Selector5/2 -> Demux8/1  "<d_xyz>"
  Bus Selector5/1 -> Demux9/1  "<xyz>"
  ref/1 -> Bus Selector5/1
  ref2/1 -> Bus Selector/1
  state/1 -> Bus Selector1/1
  Bus Selector/1 -> Demux5/1  "<xi_d>"
  statej/1 -> Bus Selector2/1
  Bus Selector2/1 -> Demux1/1  "<xyz>"
  Demux4/1 -> MATLAB Function2/1(xi), MATLAB Function/1(xi)
  Demux4/2 -> MATLAB Function2/2(yi), MATLAB Function/2(yi)
  Demux1/1 -> MATLAB Function/3(xj)
  Demux1/2 -> MATLAB Function/4(yj)
  Discrete-Time Integrator1/1 -> MATLAB Function1/2(phiAlpha_int)
  MATLAB Function2/1(U) -> MATLAB Function1/3(ui_gamma)
  statek/1 -> Bus Selector3/1
  Demux3/1 -> MATLAB Function/5(xk)
  Demux3/2 -> MATLAB Function/6(yk)
  Bus Selector3/1 -> Demux3/1  "<xyz>"
  MATLAB Function/1(phiAlpha) -> Scope1/1, MATLAB Function1/1(phiAlpha), Discrete-Time Integrator1/1
  Demux4/3 -> Terminator/1, MATLAB Function2/3(zi)
  Demux3/3 -> Terminator2/1
  MATLAB Function1/1(Ui_pos) -> Saturation/1
  Demux1/3 -> Terminator1/1
  statek1/1 -> Bus Selector4/1
  Demux7/1 -> MATLAB Function/7(xl)
  Demux7/2 -> MATLAB Function/8(yl)
  Demux7/3 -> Terminator3/1
  Bus Selector4/1 -> Demux7/1  "<xyz>"
  Bus Selector1/1 -> Demux4/1  "<xyz>"
  [yaw3] -> MATLAB Function1/4(yaw)
  MATLAB Function1/2(ui_yaw) -> Saturation1/1
  [K_con] -> MATLAB Function2/19(K_cts)
  MATLAB Function1/3(eyaw) -> Discrete-Time Integrator3/1, Memory/1
  [K_alpha] -> MATLAB Function1/6(KP)
  [params] -> MATLAB Function/9(params)
  [S_con] -> MATLAB Function2/20(S_cts)
  Bus Selector/2 -> Demux2/1  "<dxi_d>"
  [eyaw1] -> MATLAB Function1/7(eyaw1)
  [eyaw2] -> MATLAB Function1/8(eyaw2)
  Memory/1 -> [eyaw3]
  Discrete-Time Integrator3/1 -> MATLAB Function1/5(ieyaw)
  MATLAB Function2/3(S) -> To Workspace7/1, Scope2/1
  Saturation/1 -> U_ipos/1
  Saturation1/1 -> U_iyaw/1
  Bus Selector1/2 -> [d_xyz]  "<d_xyz>"
  Demux6/1 -> MATLAB Function2/4(dxi)
  Demux6/2 -> MATLAB Function2/5(dyi)
  Demux6/3 -> MATLAB Function2/6(dzi)
  [d_xyz] -> Demux6/1

== matlab function test_sliding_formation_gazebo_aerospace23a/Virtual_leader ==
  data: t input; xi_d output; dxi_d output; Xd input; f input
function [xi_d, dxi_d]  = fcn(t, Xd, f)
%#codegen



%f=1/100;    %freq in Hz
radius= 0.275;   %radius in meters 0.15
sel=1;      %inputs or parameters dont work! only local vars ...

if sel == 1
    if t < 30
       xd     =  0;
       xdotd  =  0;
           
       yd     = 0;
       ydotd  = 0;
           
       zd     = 1;  
       zdotd  = 0; 
           
       xi_d =[xd; yd; zd];
       dxi_d=[xdotd; ydotd; zdotd]; 
       
    % elseif t < 70
    %     xd     =  0.4;
    %     xdotd  =  0;
    % 
    %     yd     = -0.4;
    %     ydotd  = 0;
    % 
    %     zd     = 2.5;  
    %     zdotd  = 0; 
    % 
    %     xi_d =[xd; yd; zd];
    %     dxi_d=[xdotd; ydotd; zdotd]; 
        
    elseif t < 120  %140
       xd     = 0.1 + radius*sin(2*pi*f*t);
       xdotd  = radius*2*pi*f*cos(2*pi*f*t);
            
       yd     = 0.15 + radius*cos(2*pi*f*t);
       ydotd  = -radius*2*pi*f*sin(2*pi*f*t);
            
       zd     = 1.2; %0.2*cos(2*pi*f*t) + 1;
       zdotd  = 0; %-0.2*2*pi*f*sin(2*pi*f*t);
           
       xi_d =[xd; yd; zd];
       dxi_d=[xdotd; ydotd; zdotd];
    else
        xd     =  -0.2;
        xdotd  =  0;
            
        yd     = 0.1;
        ydotd  = 0;
            
        zd     = 1.1;  
        zdotd  = 0; 
            
        xi_d =[xd; yd; zd];
        dxi_d=[xdotd; ydotd; zdotd];        
    end
end

 if(sel==2)
     xd     =  Xd(1);
     xdotd  =  0;
          
     yd     = Xd(2);
     ydotd  = 0;
          
     zd     = Xd(3);  
     zdotd  = 0; 
          
     xi_d =[xd; yd; zd];
     dxi_d=[xdotd; ydotd; zdotd]; 
     
 end

== matlab function test_sliding_formation_gazebo_aerospace23a/Translational Control2/Flocking1/MATLAB Function ==
  data: xi input; yi input; phiAlpha output; xj input; yj input; xk input; yk input; xl input; yl input; params input

function phiAlpha  = phiAlphaFcn(xi, yi, xj, yj, xk, yk, xl, yl, params)
    
    % Flocking parameters
    epsilon = params(1); a = params(2); b = params(3); c = params(4); d = params(5); h = params(6);

    e = abs(a - b) / sqrt(4*a*b) ;

    cAlpha = sigmaNormFun(c, epsilon) ;
    dAlpha = sigmaNormFun(d, epsilon) ;

    %%
    Pi = [xi;yi] ;
    Pj = [xj;yj] ;
    Pk = [xk;yk] ;
    Pl = [xl;yl] ;

    %%
    sigmaNormj = sigmaNormFun(Pj - Pi, epsilon) ;
    nij = gradSigmaFun(Pj - Pi, epsilon) ;
    
    sigmaNormk = sigmaNormFun(Pk - Pi, epsilon) ;
    nik = gradSigmaFun(Pk - Pi, epsilon) ;

    sigmaNorml = sigmaNormFun(Pl - Pi, epsilon) ;
    nil = gradSigmaFun(Pl - Pi, epsilon) ;

    %%
    sigma1j = sigma1Fun(sigmaNormj - dAlpha + e) ;
    sigma1k = sigma1Fun(sigmaNormk - dAlpha + e) ;
    sigma1l = sigma1Fun(sigmaNorml - dAlpha + e) ;
            
    %% Position
    phiAlphaj = 0.5 * bumpFcn(sigmaNormj/cAlpha,h) * ((a+b)*sigma1j + (a-b)) ;
    phiAlphanij = phiAlphaj.* nij ;
    
    phiAlphak = 0.5 * bumpFcn(sigmaNormk/cAlpha,h) * ((a+b)*sigma1k + (a-b)) ;
    phiAlphanik = phiAlphak.* nik ;

    phiAlphal = 0.5 * bumpFcn(sigmaNorml/cAlpha,h) * ((a+b)*sigma1l + (a-b)) ;
    phiAlphanil = phiAlphal.* nil ;

    phiAlpha = phiAlphanij + phiAlphanik + phiAlphanil;

    
end

== matlab function test_sliding_formation_gazebo_aerospace23a/Translational Control2/Flocking1/MATLAB Function1 ==
  data: phiAlpha input; phiAlpha_int input; ui_gamma input; yaw input; ieyaw input; Ui_pos output size=3; ui_yaw output; KP input; eyaw output; eyaw1 input; eyaw3 input

function [Ui_pos, ui_yaw, eyaw]  = ctrlLaw(phiAlpha, phiAlpha_int, ui_gamma, yaw, ieyaw, KP, eyaw1, eyaw3)  
    
    % Control gains and parameters
    Kx = KP(1); Ky = KP(2); Kz = KP(3);
    Kix = KP(4); Kiy = KP(5); Kiz = KP(6);
    Kyaw = KP(7); Kdyaw = KP(8); Kiyaw = KP(9);
    offset = KP(10);
    
    eyaw = 0 - yaw(1);
    deyaw = 0 - yaw(2);

    ui_yaw = Kyaw*eyaw + Kdyaw*deyaw + Kiyaw*ieyaw;
    hz_dot = ui_gamma(3,1);  %

    if eyaw < offset && eyaw > -offset && eyaw1 < offset && eyaw1 > -offset && eyaw3 < offset && eyaw3 > -offset 
        hx_dot =  ui_gamma(1,1);  %Kx * phiAlpha(1,1) + Kix * phiAlpha_int(1,1) + 
        hy_dot =  ui_gamma(2,1);  %Ky * phiAlpha(2,1) + Kiy * phiAlpha_int(2,1) + 
    else
        hx_dot =  0;  %
        hy_dot =  0;  %
    end    

    Ui_pos = [hx_dot; hy_dot; hz_dot] ;
    

end

== matlab function test_sliding_formation_gazebo_aerospace23a/Translational Control2/Flocking1/MATLAB Function2 ==
  data: xi input; yi input; zi input; dxi input; dyi input; dzi input; U output; ep output; xr input; yr input; zr input; dxr input; dyr input; dzr input; xr2 input; yr2 input; zr2 input; dxr2 input; dyr2 input; dzr2 input; S output; K_cts input; S_cts input

function [U, ep, S] = naviFeedback(xi, yi, zi, dxi, dyi, dzi, xr, yr, zr, dxr, dyr, dzr, xr2, yr2, zr2, dxr2, dyr2, dzr2, K_cts, S_cts)
    
    Kp = K_cts(1); Ki = K_cts(2); Kpz = K_cts(3);

    % Cts manifold
    a_xy = S_cts(1); b_xy = S_cts(2); lam_xy = S_cts(3); p_xy = S_cts(4); q_xy= S_cts(5);
    a_z = S_cts(6); b_z = S_cts(7); lam_z = S_cts(8); p_z = S_cts(9); q_z= S_cts(10);
    
    %errors
    ex = (xr - xi - 0.75) + (xr2 - xi - 0.25);
    ey = (yr - yi - 0.43) + (yr2 - yi - 0.43);
    ez = (zr - zi) + (zr2 - zi);
    ep = [ex;ey;ez];

    dex = (dxr - dxi) + (dxr2 - dxi);
    dey = (dyr - dyi) + (dyr2 - dyi);
    dez = (dzr - dzi) + (dzr2 - dzi);
    
    %Manifold definitions
    Sx = ex;
    Sy = ey;
    Sz = ez;

    S = [Sx;Sy;Sz];

    ux = dxr+dxr2 + Kp*tanh(Sx) ;
    uy = dyr+dyr2 + Kp*tanh(Sy);
    uz = dzr+dzr2 + Kpz*tanh(Sz);

    U = [ux;uy;uz];
end

== matlab function test_sliding_formation_gazebo_aerospace23a/Translational Control3/Flocking1/MATLAB Function ==
  data: xi input; yi input; phiAlpha output; xj input; yj input; xk input; yk input; xl input; yl input; params input

function phiAlpha  = phiAlphaFcn(xi, yi, xj, yj, xk, yk, xl, yl, params)
    
    % Flocking parameters
    epsilon = params(1); a = params(2); b = params(3); c = params(4); d = params(5); h = params(6);

    e = abs(a - b) / sqrt(4*a*b) ;

    cAlpha = sigmaNormFun(c, epsilon) ;
    dAlpha = sigmaNormFun(d, epsilon) ;

    %%
    Pi = [xi;yi] ;
    Pj = [xj;yj] ;
    Pk = [xk;yk] ;
    Pl = [xl;yl] ;

    %%
    sigmaNormj = sigmaNormFun(Pj - Pi, epsilon) ;
    nij = gradSigmaFun(Pj - Pi, epsilon) ;
    
    sigmaNormk = sigmaNormFun(Pk - Pi, epsilon) ;
    nik = gradSigmaFun(Pk - Pi, epsilon) ;

    sigmaNorml = sigmaNormFun(Pl - Pi, epsilon) ;
    nil = gradSigmaFun(Pl - Pi, epsilon) ;

    %%
    sigma1j = sigma1Fun(sigmaNormj - dAlpha + e) ;
    sigma1k = sigma1Fun(sigmaNormk - dAlpha + e) ;
    sigma1l = sigma1Fun(sigmaNorml - dAlpha + e) ;
            
    %% Position
    phiAlphaj = 0.5 * bumpFcn(sigmaNormj/cAlpha,h) * ((a+b)*sigma1j + (a-b)) ;
    phiAlphanij = phiAlphaj.* nij ;
    
    phiAlphak = 0.5 * bumpFcn(sigmaNormk/cAlpha,h) * ((a+b)*sigma1k + (a-b)) ;
    phiAlphanik = phiAlphak.* nik ;

    phiAlphal = 0.5 * bumpFcn(sigmaNorml/cAlpha,h) * ((a+b)*sigma1l + (a-b)) ;
    phiAlphanil = phiAlphal.* nil ;

    phiAlpha = phiAlphanij + phiAlphanik + phiAlphanil;

    
end

== matlab function test_sliding_formation_gazebo_aerospace23a/Translational Control3/Flocking1/MATLAB Function1 ==
  data: phiAlpha input; phiAlpha_int input; ui_gamma input; yaw input; ieyaw input; Ui_pos output size=3; ui_yaw output; KP input; eyaw output; eyaw1 input; eyaw2 input

function [Ui_pos, ui_yaw, eyaw]  = ctrlLaw(phiAlpha, phiAlpha_int, ui_gamma, yaw, ieyaw, KP, eyaw1, eyaw2)  
    
    % Control gains and parameters
    Kx = KP(1); Ky = KP(2); Kz = KP(3);
    Kix = KP(4); Kiy = KP(5); Kiz = KP(6);
    Kyaw = KP(7); Kdyaw = KP(8); Kiyaw = KP(9);
    offset = KP(10);
    
    eyaw = 0 - yaw(1);
    deyaw = 0 - yaw(2);

    ui_yaw = Kyaw*eyaw + Kdyaw*deyaw + Kiyaw*ieyaw;
    hz_dot = ui_gamma(3,1);  %

    if eyaw < offset && eyaw > -offset && eyaw1 < offset && eyaw1 > -offset && eyaw2 < offset && eyaw2 > -offset 
        hx_dot =  ui_gamma(1,1);  %Kx * phiAlpha(1,1) + Kix * phiAlpha_int(1,1) + 
        hy_dot =  ui_gamma(2,1);  %Ky * phiAlpha(2,1) + Kiy * phiAlpha_int(2,1) + 
    else
        hx_dot =  0;  %
        hy_dot =  0;  %
    end    

    Ui_pos = [hx_dot; hy_dot; hz_dot] ;
    

end

== matlab function test_sliding_formation_gazebo_aerospace23a/Translational Control3/Flocking1/MATLAB Function2 ==
  data: xi input; yi input; zi input; dxi input; dyi input; dzi input; U output; xr input; yr input; zr input; dxr input; dyr input; dzr input; xr2 input; yr2 input; zr2 input; dxr2 input; dyr2 input; dzr2 input; ep output size=3; S output; K_cts input; S_cts input

function [U, ep, S] = naviFeedback(xi, yi, zi, dxi, dyi, dzi, xr, yr, zr, dxr, dyr, dzr, xr2, yr2, zr2, dxr2, dyr2, dzr2, K_cts, S_cts)
    
    Kp = K_cts(1); Ki = K_cts(2); Kpz = K_cts(3);

    % Cts manifold
    a_xy = S_cts(1); b_xy = S_cts(2); lam_xy = S_cts(3); p_xy = S_cts(4); q_xy= S_cts(5);
    a_z = S_cts(6); b_z = S_cts(7); lam_z = S_cts(8); p_z = S_cts(9); q_z= S_cts(10);
    
    %errors
    ex = (xr - xi) + (xr2 - xi - 0.25);
    ey = (yr - yi + 0.86) + (yr2 - yi + 0.43);
    ez = (zr - zi) + (zr2 - zi);
    ep = [ex;ey;ez];

    dex = (dxr - dxi) + (dxr2 - dxi);
    dey = (dyr - dyi) + (dyr2 - dxi);
    dez = (dzr - dzi) + (dzr2 - dxi);
    E = [ex;ey;ez;dex;dey;dez];

    %Manifold definitions
    Sx = ex;
    Sy = ey;
    Sz = ez;

    S = [Sx;Sy;Sz];

    ux = dxr+dxr2 + Kp*tanh(Sx) ;
    uy = dyr+dyr2 + Kp*tanh(Sy);
    uz = dzr+dzr2 + Kpz*tanh(Sz);

    U = [ux;uy;uz];
end

== matlab function test_sliding_formation_gazebo_aerospace23a/Extract pose 1/Observer_for_speed ==
  data: X input; dXhat_1 output; Xhat input; Xhat2 input; K1ob input; K2ob input; dXhat_2 output
function [dXhat_1, dXhat_2] = fcn(X, Xhat, Xhat2, K1ob, K2ob)

%%
%Separation of the actual states
X_a = X(1:3);
x = X_a(1);  y = X_a(2);  z = X_a(3);    

%%
%Estimation vector separation
X_hat = Xhat(1:3);
x_h1 = X_hat(1);
y_h1 = X_hat(2);
z_h1 = X_hat(3);

%%
%Observer errors definition
e_x = x - x_h1;
e_y = y - y_h1;
e_z = z - z_h1;

%%
%Vector form
e_X = [e_x;e_y;e_z];

pow = [0.5;0.5;0.5];

%%
%Computation of the observer
dXhat_1 = Xhat2 + (K1ob*abs(e_X).^pow).*tanh(e_X);
dXhat_2 = K2ob*tanh(e_X);

== matlab function test_sliding_formation_gazebo_aerospace23a/Translational Control1/Flocking1/MATLAB Function ==
  data: xi input; yi input; phiAlpha output; xj input; yj input; xk input; yk input; xl input; yl input; params input

function phiAlpha  = phiAlphaFcn(xi, yi, xj, yj, xk, yk, xl, yl, params)
    
    % Flocking parameters
    epsilon = params(1); a = params(2); b = params(3); c = params(4); d = params(5); h = params(6);

    e = abs(a - b) / sqrt(4*a*b) ;

    cAlpha = sigmaNormFun(c, epsilon) ;
    dAlpha = sigmaNormFun(d, epsilon) ;

    %%
    Pi = [xi;yi] ;
    Pj = [xj;yj] ;
    Pk = [xk;yk] ;
    Pl = [xl;yl] ;

    %%
    sigmaNormj = sigmaNormFun(Pj - Pi, epsilon) ;
    nij = gradSigmaFun(Pj - Pi, epsilon) ;
    
    sigmaNormk = sigmaNormFun(Pk - Pi, epsilon) ;
    nik = gradSigmaFun(Pk - Pi, epsilon) ;

    sigmaNorml = sigmaNormFun(Pl - Pi, epsilon) ;
    nil = gradSigmaFun(Pl - Pi, epsilon) ;

    %%
    sigma1j = sigma1Fun(sigmaNormj - dAlpha + e) ;
    sigma1k = sigma1Fun(sigmaNormk - dAlpha + e) ;
    sigma1l = sigma1Fun(sigmaNorml - dAlpha + e) ;
            
    %% Position
    phiAlphaj = 0.5 * bumpFcn(sigmaNormj/cAlpha,h) * ((a+b)*sigma1j + (a-b)) ;
    phiAlphanij = phiAlphaj.* nij ;
    
    phiAlphak = 0.5 * bumpFcn(sigmaNormk/cAlpha,h) * ((a+b)*sigma1k + (a-b)) ;
    phiAlphanik = phiAlphak.* nik ;

    phiAlphal = 0.5 * bumpFcn(sigmaNorml/cAlpha,h) * ((a+b)*sigma1l + (a-b)) ;
    phiAlphanil = phiAlphal.* nil ;

    phiAlpha = phiAlphanij + phiAlphanik + phiAlphanil;

    
end

== matlab function test_sliding_formation_gazebo_aerospace23a/Translational Control1/Flocking1/MATLAB Function1 ==
  data: phiAlpha input; phiAlpha_int input; ui_gamma input; yaw input; ieyaw input; Ui_pos output size=3; ui_yaw output; KP input; eyaw output; eyaw2 input; eyaw3 input

function [Ui_pos, ui_yaw, eyaw]  = ctrlLaw(phiAlpha, phiAlpha_int, ui_gamma, yaw, ieyaw, KP, eyaw2, eyaw3)  
    
    % Control gains and parameters
    Kx = KP(1); Ky = KP(2); Kz = KP(3);
    Kix = KP(4); Kiy = KP(5); Kiz = KP(6);
    Kyaw = KP(7); Kdyaw = KP(8); Kiyaw = KP(9);
    offset = KP(10);
    
    eyaw = 0 - yaw(1);
    deyaw = 0 - yaw(2);

    ui_yaw = Kyaw*eyaw + Kdyaw*deyaw + Kiyaw*ieyaw;
    hz_dot = ui_gamma(3,1);  %

    if eyaw < offset && eyaw > -offset && eyaw2 < offset && eyaw2 > -offset && eyaw3 < offset && eyaw3 > -offset 
        hx_dot =  ui_gamma(1,1);  %Kx * phiAlpha(1,1) + Kix * phiAlpha_int(1,1) + 
        hy_dot =  ui_gamma(2,1);  %Ky * phiAlpha(2,1) + Kiy * phiAlpha_int(2,1) + 
    else
        hx_dot =  0;  %
        hy_dot =  0;  %
    end    

    Ui_pos = [hx_dot; hy_dot; hz_dot] ;
    

end

== matlab function test_sliding_formation_gazebo_aerospace23a/Translational Control1/Flocking1/MATLAB Function2 ==
  data: xi input; yi input; zi input; dxi input; dyi input; dzi input; U output; xr input; yr input; zr input; dxr input; dyr input; dzr input; S output; K_cts input; S_cts input

function [U, S] = naviFeedback(xi, yi, zi, dxi, dyi, dzi, xr, yr, zr, dxr, dyr, dzr, K_cts, S_cts)
    
    Kp = K_cts(1); Ki = K_cts(2); Kpz = K_cts(3);

    % Cts manifold
    a_xy = S_cts(1); b_xy = S_cts(2); lam_xy = S_cts(3); p_xy = S_cts(4); q_xy= S_cts(5);
    a_z = S_cts(6); b_z = S_cts(7); lam_z = S_cts(8); p_z = S_cts(9); q_z= S_cts(10);
    
    %errors
    ex = (xr - xi + 0.5);
    ey = (yr - yi);
    ez = (zr - zi);
    ep = [ex;ey;ez];

    dex = (dxr - dxi);
    dey = (dyr - dyi);
    dez = (dzr - dzi);
    
    %Manifold definitions
    Sx = ex;
    Sy = ey;
    Sz = ez;

    S = [Sx;Sy;Sz];

    ux = dxr + Kp*tanh(Sx) ;
    uy = dyr + Kp*tanh(Sy);
    uz = dzr + Kpz*tanh(Sz);

    U = [ux;uy;uz];
end

== matlab function test_sliding_formation_gazebo_aerospace23a/Extract pose 2/Observer_for_speed ==
  data: X input; dXhat_1 output; Xhat input; Xhat2 input; K1ob input; K2ob input; dXhat_2 output
function [dXhat_1, dXhat_2] = fcn(X, Xhat, Xhat2, K1ob, K2ob)

%%
%Separation of the actual states
X_a = X(1:3);
x = X_a(1);  y = X_a(2);  z = X_a(3);    

%%
%Estimation vector separation
X_hat = Xhat(1:3);
x_h1 = X_hat(1);
y_h1 = X_hat(2);
z_h1 = X_hat(3);

%%
%Observer errors definition
e_x = x - x_h1;
e_y = y - y_h1;
e_z = z - z_h1;

%%
%Vector form
e_X = [e_x;e_y;e_z];

pow = [0.5;0.5;0.5];

%%
%Computation of the observer
dXhat_1 = Xhat2 + (K1ob*abs(e_X).^pow).*tanh(e_X);
dXhat_2 = K2ob*tanh(e_X);

== matlab function test_sliding_formation_gazebo_aerospace23a/Extract pose 3/Observer_for_speed ==
  data: X input; dXhat_1 output; Xhat input; Xhat2 input; K1ob input; K2ob input; dXhat_2 output
function [dXhat_1, dXhat_2] = fcn(X, Xhat, Xhat2, K1ob, K2ob)

%%
%Separation of the actual states
X_a = X(1:3);
x = X_a(1);  y = X_a(2);  z = X_a(3);    

%%
%Estimation vector separation
X_hat = Xhat(1:3);
x_h1 = X_hat(1);
y_h1 = X_hat(2);
z_h1 = X_hat(3);

%%
%Observer errors definition
e_x = x - x_h1;
e_y = y - y_h1;
e_z = z - z_h1;

%%
%Vector form
e_X = [e_x;e_y;e_z];

pow = [0.5;0.5;0.5];

%%
%Computation of the observer
dXhat_1 = Xhat2 + (K1ob*abs(e_X).^pow).*tanh(e_X);
dXhat_2 = K2ob*tanh(e_X);
